simulink model "Fuzzy_2409_1"  (R2018a)
settings: Solver=VariableStepAuto  StartTime=0.0  StopTime=20  RelTol=1e-6  EnableMultiTasking=on
undefined symbols (not defined in the file): sigbuilder_block
libraries: fuzblock x1
settings Model: Creator=USER  LastModifiedBy=forev
settings OptimizationCC: LifeSpan=inf
settings DebuggingCC: SFUnexpectedBacktrackingDiag=warning  SFNoUnconditionalDefaultTransitionDiag=warning  SFExecutionAtInitializationDiag=none
settings CodeAppCC: StateflowObjectComments=on
settings GRTTargetCC: TargetLangStandard=C89/C90 (ANSI)  GeneratePreprocessorConditionals=Disable all
settings ConfigComp: CovMetricSettings=dw  CovHtmlReporting=on  CovSaveCumulativeToWorkspaceVar=on  CovSaveSingleToWorkspaceVar=on  CovExternalEMLEnable=off

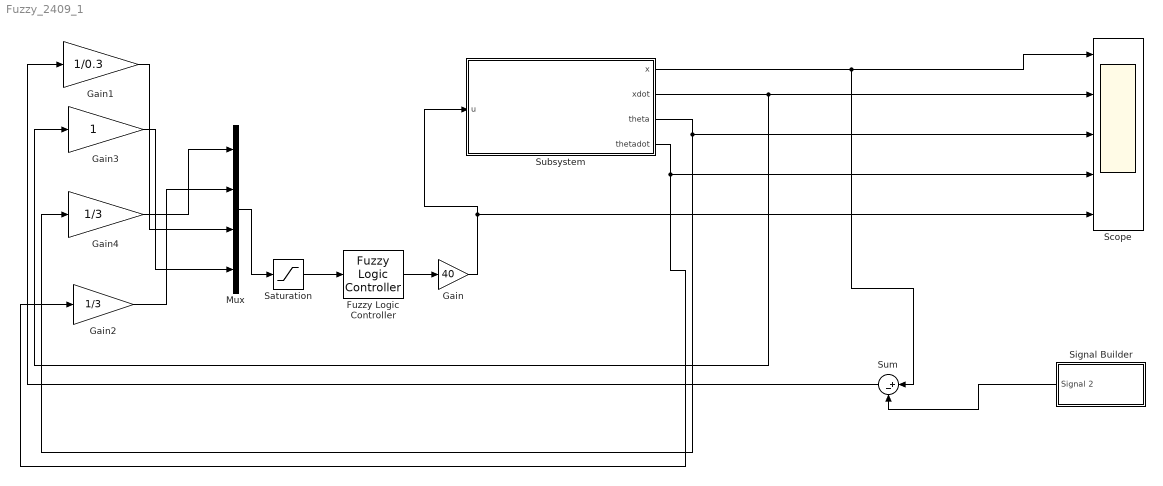
== system Fuzzy_2409_1 ==
  Fuzzy Logic Controller : fuzblock/Fuzzy Logic  Controller  FIS=['fuzzy_rule.fis']  OutputSampleNumber=101  DataType=double  FuzzifiedInputs=off  RuleFiringStrengths=off  RuleOutputs=off  AggregatedOutputs=off  SimulateUsing=Interpreted execution  OutOfRangeInputValueMessage=warning  NoRuleFiredMessage=warning  EmptyOutputFuzzySetMessage=warning
  Gain : Gain  Gain=40
  Gain1 : Gain  Gain=1/0.3
  Gain2 : Gain  Gain=1/3
  Gain3 : Gain
  Gain4 : Gain  Gain=1/3
  Mux : Mux
  Saturation : Saturate  UpperLimit=1  LowerLimit=-1
  Scope : Scope  NumInputPorts=5
  Signal Builder : Subsystem  Tag=STV Subsys  LoadFcn=sigbuilder_block('load');  StartFcn=sigbuilder_block('start');  StopFcn=sigbuilder_block('stop');  ClipboardFcn=sigbuilder_block('clipboard');  mask(Sigbuilder block){tuvar=[0:10]}
      mask help: Simulink:masks:SigbuilderBlock_MD
      mask init:
      | if ~strcmp(get_param(bdroot(gcbh),'SimulationStatus'),'stopped') tuvar = sigbuilder_block('maskInit'); end
      settings: CopyFcn=sigbuilder_block('copy');  DeleteFcn=sigbuilder_block('delete');  ModelCloseFcn=sigbuilder_block('modelClose');  PreSaveFcn=sigbuilder_block('preSave');  PauseFcn=sigbuilder_block('pause');  ContinueFcn=sigbuilder_block('continue');  NameChangeFcn=sigbuilder_block('namechange');  OpenFcn=sigbuilder_block('open',[437.4 199.2 550.8 400.2 ]);  CloseFcn=sigbuilder_block('close');
      mask Display: plot(0, 0, 100, 100,[2, 2, 32, 32, 2], [68, 8, 8, 68, 68],[32, 2], [38, 38], [32, 19, 2],[53, 60, 44], [32, 17, 17, 2],[16, 16, 31, 31]);txt = getActiveGroup(gcbh);text(2, 100, txt,'verticalAlignment', 'top');
  Subsystem : Subsystem  mask{l=0.5, k=0.1, M=1, g=9.81, y0=pi/4, ydot0=pi, x0=0.5, xdot0=0.5}
      mask prompts: l "chieu dai"; k "Khoi luong"; M "khoi luong 2"; g "gia toc tt"; y0 "goc ban dau"; ydot0 "vt goc ban dau"; x0 "vi tri x ban dau"; xdot0 "vi tri xdot ban dau"
  Sum : Sum  Inputs=|+-
  wires:
  Mux/1 -> Saturation/1
  Saturation/1 -> Fuzzy Logic Controller/1
  Fuzzy Logic Controller/1 -> Gain/1
  Gain/1 -> Scope/5, Subsystem/1(u)
  Subsystem/1("x ") -> Sum/1, Scope/1
  Subsystem/2("xdot ") -> Gain3/1, Scope/2
  Subsystem/3(theta) -> Scope/3, Gain4/1
  Subsystem/4(thetadot) -> Gain2/1, Scope/4
  Signal Builder/1(Signal 2) -> Sum/2
  Sum/1 -> Gain1/1
  Gain4/1 -> Mux/1
  Gain2/1 -> Mux/2
  Gain3/1 -> Mux/4
  Gain1/1 -> Mux/3

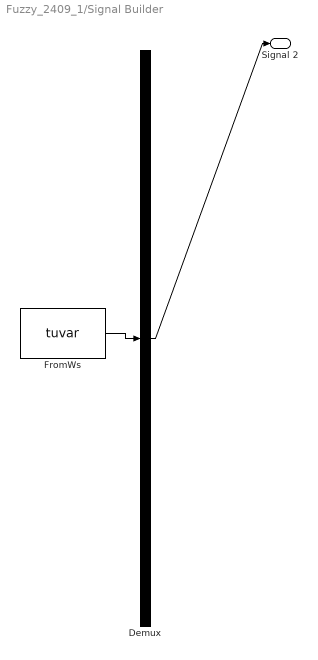
== system Fuzzy_2409_1/Signal Builder ==
  Demux : Demux  Tag=STV Demux  Outputs=1
  FromWs : FromWorkspace  Tag=STV FromWs  VariableName=tuvar  SampleTime=0
      SigBuilderData=|
      | common.afterFinalStr = 'Extrapolate'
      | common.sampleTime = 0
      | dataSet.timeRange = [0 20]
      | dataSet.name = 'Group 1'
      | sbobj.Groups.Name = 'Group 1'
      | sbobj.Groups.Signals.Name = 'Signal 2'
      | sbobj.Groups.Signals.XData = [0 10.05 10.05 20]
      | sbobj.Groups.Signals.YData = [1 1 0 0]
      | sbobj.Groups.TimeRange = [0 20]
  Signal 2 : Outport  Tag=STV Outport
  wires:
  FromWs/1 -> Demux/1
  Demux/1 -> Signal 2/1

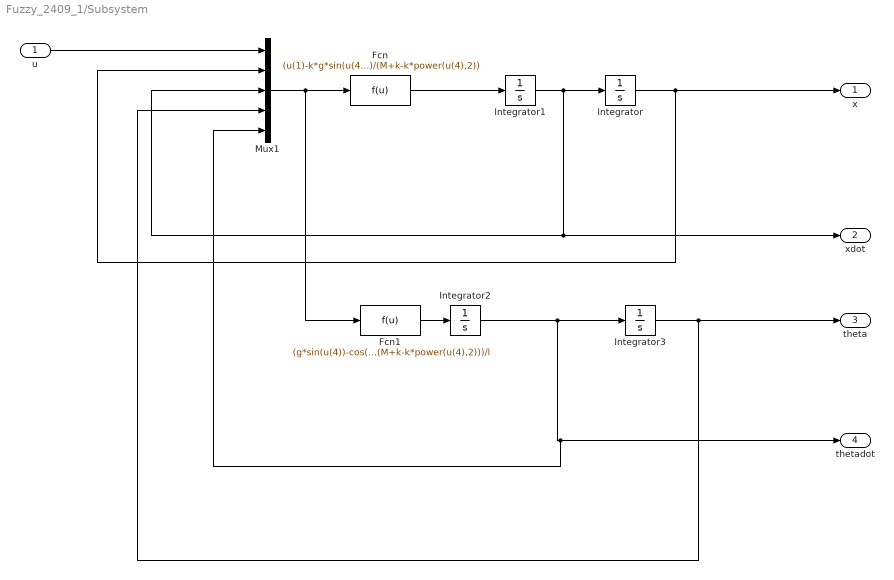
== system Fuzzy_2409_1/Subsystem ==
  u : Inport
  Fcn : Fcn  Expr=(u(1)-k*g*sin(u(4))*cos(u(4))+k*l*sin(u(4))*power(u(5),2))/(M+k-k*power(u(4),2))
  Fcn1 : Fcn  Expr=(g*sin(u(4))-cos(u(4))*(u(1)-k*g*sin(u(4))*cos(u(4))+k*l*sin(u(4))*power(u(5),2))/(M+k-k*power(u(4),2)))/l
  Integrator : Integrator  InitialCondition=ydot0
  Integrator1 : Integrator  InitialCondition=y0
  Integrator2 : Integrator  InitialCondition=x0
  Integrator3 : Integrator  InitialCondition=xdot0
  Mux1 : Mux  Inputs=5
  "x " : Outport
  "xdot " : Outport  Port=2
  theta : Outport  Port=3
  thetadot : Outport  Port=4
  wires:
  Integrator/1 -> Mux1/2, "x "/1
  Fcn/1 -> Integrator1/1
  Integrator1/1 -> Mux1/3, "xdot "/1, Integrator/1
  Integrator2/1 -> Mux1/5, thetadot/1, Integrator3/1
  Integrator3/1 -> Mux1/4, theta/1
  Mux1/1 -> Fcn1/1, Fcn/1
  Fcn1/1 -> Integrator2/1
  u/1 -> Mux1/1
